simulink model "platoon_model"  (R2024a)
settings: Solver=VariableStepAuto  StartTime=0.0  StopTime=150  RelTol=1e-3
values from neighbouring files (symbols this model uses):
  d_0 = 8    [platoon.m]
  Kd_err = parameter_sets{i}.Kd_err    [platoon.m]
  Kv = parameter_sets{i}.Kv    [platoon.m]
  Kv_r = parameter_sets{i}.Kd_r    [platoon.m]
  t_h_tar = 1    [platoon.m]
  v_initial = v_initial_params{i}    [platoon.m]
  v_tar = 30    [platoon.m]
  x_initial = [150 100 50 0]    [platoon.m]
libraries: simulink x8
settings Model: Creator=alessandro  LastModifiedBy=vaidh
settings SolverCC: AlgebraicLoopSolver=TrustRegion
settings DebuggingCC: UnconnectedInputMsg=warning  UnconnectedOutputMsg=warning  UnconnectedLineMsg=warning
settings ModelReferenceCC: EnableRefExpFcnMdlSchedulingChecks=on
settings RTWCC: GPUComputeCapability=3.5  DLArmComputeVersion=19.05

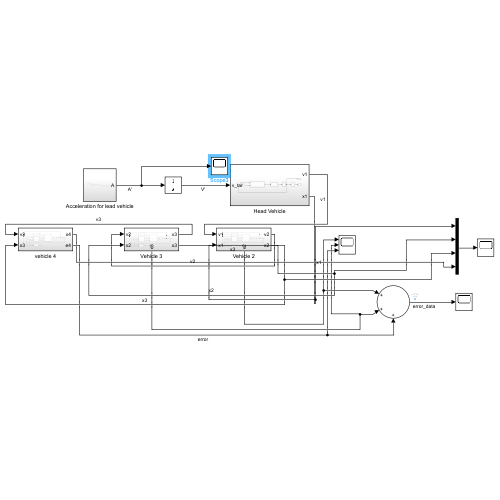
[thumbnail: Simulink's stored preview of the top-level diagram]
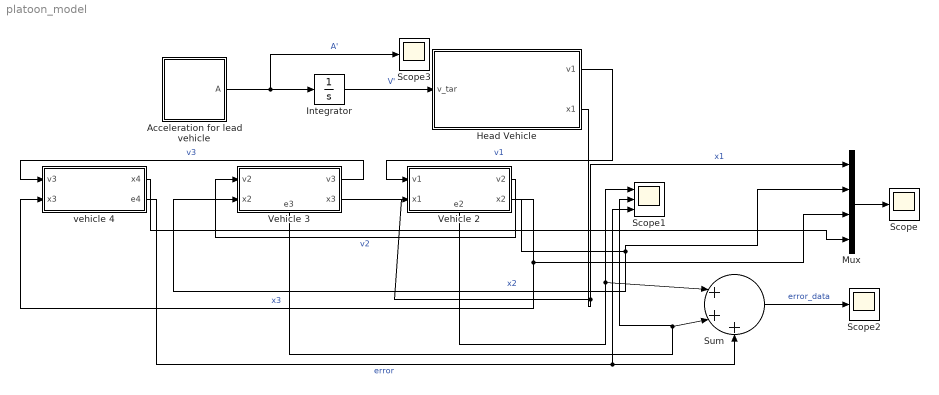
== system platoon_model ==
  Acceleration for lead vehicle : Subsystem
  "Head Vehicle " : Subsystem
  Integrator : Integrator  InitialCondition=v_initial(1)
  Mux : Mux
  Scope : Scope
  Scope1 : Scope  NumInputPorts=3
  Scope2 : Scope
  Scope3 : Scope
  Sum : Sum  Inputs=|+++
  Vehicle 2 : Subsystem
      settings: PortSchema="{\"entries\":[{\"content\":{\"sides\":[{\"content\":{\"connectorIds\":[\"In1\",\"In2\"]},\"type\":\"ConnectorPlacement.EquallySpacedRectSide\",\"uuid\":\"2c5fe078-c65f-41b6-8525-e64b013db54d\"},{\"content\":{\"connectorIds\":[\"Out1\",\"Out2\"],\"side\":\"RIGHT\"},\"type\":\"ConnectorPlacement.EquallySpacedRectSide\",\"uuid\":\"224ddbf7-34e7-4cd5-bbc2-438b58b736fb\"},{\"content\":{\"connectorIds\":[],\"side\":\"TOP\"},\"type\":\"ConnectorPlacement.EquallySpacedRectSide\",\"uuid\":\"73fb06e4-4483-4cd2-bdf8-037e0f1850b0\"},{\"content\":{\"connectorIds\":[\"Out3\"],\"side\":\"BOTTOM\"},\"type\":\"ConnectorPlacement.EquallySpacedRectSide\",\"uuid\":\"d300d9ad-fcb1-499a-b20a-481d5a2cf245\"},{\"content\":{\"connectorIds\":[],\"side\":\"HIDDEN\"},\"type\":\"ConnectorPlacement.EquallySpacedRectSide\",\"uuid\":\"4daeff91-7956-45e4-9a34-f5db9c954101\"}]},\"type\":\"ConnectorPlacement.EquallySpacedConnector\",\"uuid\":\"d1502d10-77ac-432c-94f4-53576a23d313\"}],\"packageUris\":[\"http://schema.mathworks.com/mf0/Connector/R2020b\"],\"version\":\"1.0\"}"
  Vehicle 3 : Subsystem
      settings: PortSchema="{\"entries\":[{\"content\":{\"sides\":[{\"content\":{\"connectorIds\":[\"In1\",\"In2\"]},\"type\":\"ConnectorPlacement.EquallySpacedRectSide\",\"uuid\":\"2c5fe078-c65f-41b6-8525-e64b013db54d\"},{\"content\":{\"connectorIds\":[\"Out1\",\"Out2\"],\"side\":\"RIGHT\"},\"type\":\"ConnectorPlacement.EquallySpacedRectSide\",\"uuid\":\"224ddbf7-34e7-4cd5-bbc2-438b58b736fb\"},{\"content\":{\"connectorIds\":[],\"side\":\"TOP\"},\"type\":\"ConnectorPlacement.EquallySpacedRectSide\",\"uuid\":\"73fb06e4-4483-4cd2-bdf8-037e0f1850b0\"},{\"content\":{\"connectorIds\":[\"Out3\"],\"side\":\"BOTTOM\"},\"type\":\"ConnectorPlacement.EquallySpacedRectSide\",\"uuid\":\"c04e4dd6-a406-4b84-b6be-e044dc5934f0\"},{\"content\":{\"connectorIds\":[],\"side\":\"HIDDEN\"},\"type\":\"ConnectorPlacement.EquallySpacedRectSide\",\"uuid\":\"4daeff91-7956-45e4-9a34-f5db9c954101\"}]},\"type\":\"ConnectorPlacement.EquallySpacedConnector\",\"uuid\":\"d1502d10-77ac-432c-94f4-53576a23d313\"}],\"packageUris\":[\"http://schema.mathworks.com/mf0/Connector/R2020b\"],\"version\":\"1.0\"}"
  vehicle 4 : Subsystem
  wires:
  Acceleration for lead vehicle/1(A) -> Scope3/1, Integrator/1  "A'"
  Integrator/1 -> "Head Vehicle "/1(v_tar)  "V'"
  "Head Vehicle "/1(v1) -> Vehicle 2/1(v1)  "v1"
  "Head Vehicle "/2(x1) -> Mux/1, Vehicle 2/2(x1)  "x1"
  Vehicle 2/1(v2) -> Vehicle 3/1(v2)  "v2"
  Vehicle 2/2(x2) -> Vehicle 3/2(x2), Mux/2  "x2"
  Vehicle 3/1(v3) -> vehicle 4/1(v3)  "v3"
  Vehicle 3/2(x3) -> vehicle 4/2(x3), Mux/3  "x3"
  vehicle 4/1(x4) -> Mux/4
  Mux/1 -> Scope/1
  Vehicle 3/3(e3) -> Sum/2, Scope1/2
  Vehicle 2/3(e2) -> Sum/1, Scope1/1
  vehicle 4/2(e4) -> Sum/3, Scope1/3  "error"
  Sum/1 -> Scope2/1  "error_data"

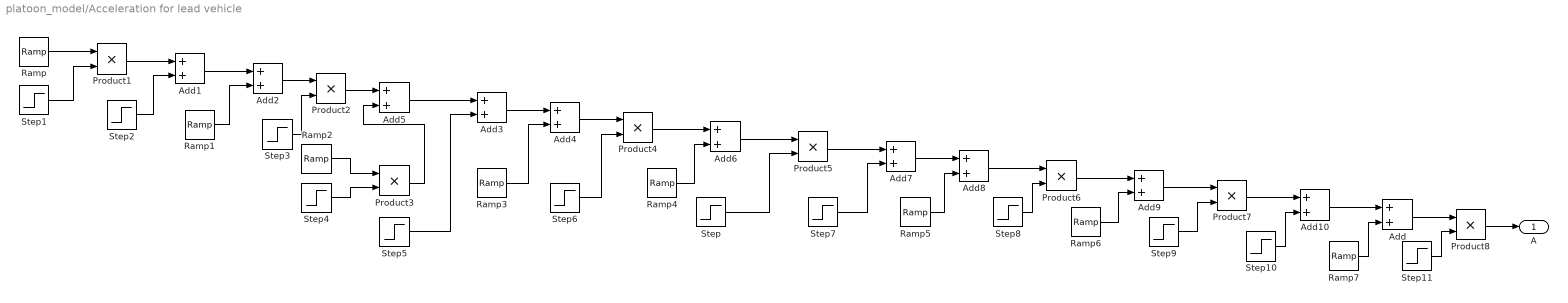
== system platoon_model/Acceleration for lead vehicle ==
  Add{,1..10} (11 alike) : Sum
  Product{1..8} (8 alike) : Product
  Ramp : simulink/Sources/Ramp  slope=-4  start=10  InitialOutput=0
  Ramp1 : simulink/Sources/Ramp  slope=4  start=13.5  InitialOutput=0
  Ramp2 : simulink/Sources/Ramp  slope=4  start=40  InitialOutput=0
  Ramp3 : simulink/Sources/Ramp  slope=-4  start=43.5  InitialOutput=0
  Ramp4 : simulink/Sources/Ramp  slope=-4  start=70  InitialOutput=0
  Ramp5 : simulink/Sources/Ramp  slope=4  start=73.5  InitialOutput=0
  Ramp6 : simulink/Sources/Ramp  slope=4  start=100  InitialOutput=0
  Ramp7 : simulink/Sources/Ramp  slope=-4  start=103.5  InitialOutput=0
  Step : Step  Time=70.5  Before=1  After=0  SampleTime=0
  Step1 : Step  Time=10.5  Before=1  After=0  SampleTime=0.1
  Step10 : Step  Time=100.5  After=2  SampleTime=0
  Step11 : Step  Time=104  Before=1  After=0  SampleTime=0
  Step2 : Step  Time=10.5  After=-2  SampleTime=0
  Step3 : Step  Time=14  Before=1  After=0  SampleTime=0
  Step4 : Step  Time=40.5  Before=1  After=0  SampleTime=0
  Step5 : Step  Time=40.5  After=2  SampleTime=0
  Step6 : Step  Time=44  Before=1  After=0  SampleTime=0
  Step7 : Step  Time=70.5  After=-2  SampleTime=0
  Step8 : Step  Time=74  Before=1  After=0  SampleTime=0
  Step9 : Step  Time=100.5  Before=1  After=0  SampleTime=0
  A : Outport
  wires:
  Add1/1 -> Add2/1
  Step3/1 -> Product2/2
  Product3/1 -> Add5/2
  Step5/1 -> Add3/2
  Add2/1 -> Product2/1
  Step1/1 -> Product1/2
  Product2/1 -> Add5/1
  Step2/1 -> Add1/2
  Ramp2/1 -> Product3/1
  Product1/1 -> Add1/1
  Add4/1 -> Product4/1
  Ramp/1 -> Product1/1
  Add3/1 -> Add4/1
  Step6/1 -> Product4/2
  Ramp1/1 -> Add2/2
  Step4/1 -> Product3/2
  Add5/1 -> Add3/1
  Ramp3/1 -> Add4/2
  Product4/1 -> Add6/1
  Ramp4/1 -> Add6/2
  Add6/1 -> Product5/1
  Step/1 -> Product5/2
  Product5/1 -> Add7/1
  Step7/1 -> Add7/2
  Add7/1 -> Add8/1
  Ramp5/1 -> Add8/2
  Add8/1 -> Product6/1
  Step8/1 -> Product6/2
  Product6/1 -> Add9/1
  Ramp6/1 -> Add9/2
  Add9/1 -> Product7/1
  Step9/1 -> Product7/2
  Step10/1 -> Add10/2
  Product7/1 -> Add10/1
  Add10/1 -> Add/1
  Ramp7/1 -> Add/2
  Add/1 -> Product8/1
  Step11/1 -> Product8/2
  Product8/1 -> A/1

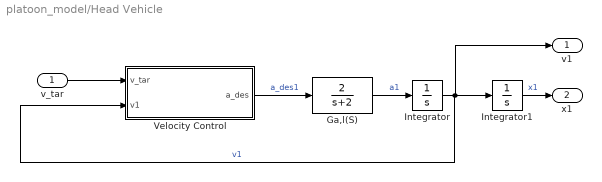
== system platoon_model/Head Vehicle  ==
  v_tar : Inport
  Ga,l(S) : TransferFcn  Numerator=[2]  Denominator=[1 2]
  Integrator : Integrator  InitialCondition=v_initial(1)
  Integrator1 : Integrator  InitialCondition=x_initial(1)
  Velocity Control : Subsystem
  v1 : Outport
  x1 : Outport  Port=2
  wires:
  Integrator/1 -> Velocity Control/2(v1), v1/1, Integrator1/1  "v1"
  Ga,l(S)/1 -> Integrator/1  "a1"
  v_tar/1 -> Velocity Control/1(v_tar)
  Velocity Control/1(a_des) -> Ga,l(S)/1  "a_des1"
  Integrator1/1 -> x1/1  "x1"

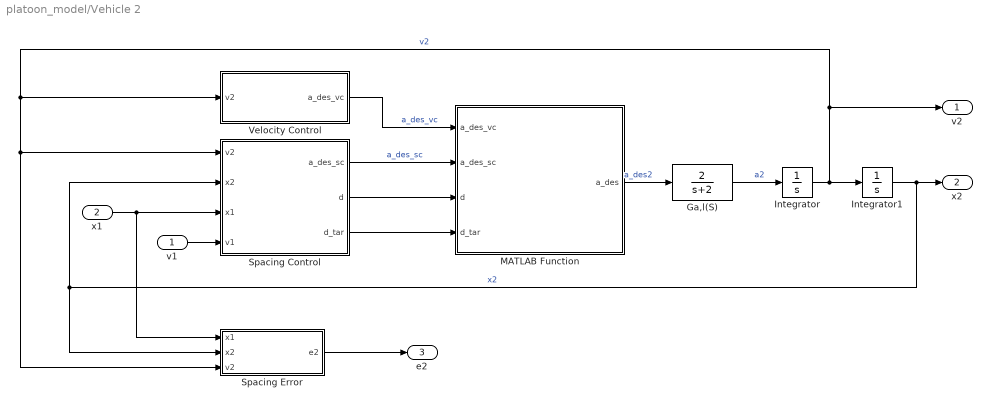
== system platoon_model/Vehicle 2 ==
  v1 : Inport
  x1 : Inport  Port=2
  Ga,l(S) : TransferFcn  Numerator=[2]  Denominator=[1 2]
  Integrator : Integrator  InitialCondition=v_initial(2)
  Integrator1 : Integrator  InitialCondition=x_initial(2)
  MATLAB Function : MATLAB Function  TreatAsAtomicUnit=on
  Spacing Control : Subsystem
  Spacing Error : Subsystem
  Velocity Control : Subsystem
  v2 : Outport
  x2 : Outport  Port=2
  e2 : Outport  Port=3
  wires:
  Spacing Control/1(a_des_sc) -> MATLAB Function/2(a_des_sc)  "a_des_sc"
  Velocity Control/1(a_des_vc) -> MATLAB Function/1(a_des_vc)  "a_des_vc"
  v1/1 -> Spacing Control/4(v1)
  x1/1 -> Spacing Control/3(x1), Spacing Error/1(x1)
  Spacing Control/2(d) -> MATLAB Function/3(d)
  MATLAB Function/1(a_des) -> Ga,l(S)/1  "a_des2"
  Integrator1/1 -> x2/1, Spacing Error/2(x2), Spacing Control/2(x2)  "x2"
  Spacing Control/3(d_tar) -> MATLAB Function/4(d_tar)
  Ga,l(S)/1 -> Integrator/1  "a2"
  Integrator/1 -> Integrator1/1, v2/1, Velocity Control/1(v2), Spacing Control/1(v2), Spacing Error/3(v2)  "v2"
  Spacing Error/1(e2) -> e2/1

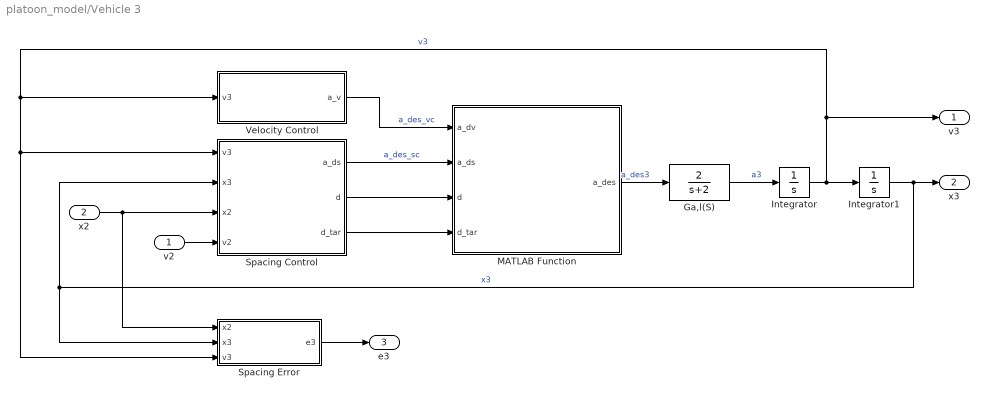
== system platoon_model/Vehicle 3 ==
  v2 : Inport
  x2 : Inport  Port=2
  Ga,l(S) : TransferFcn  Numerator=[2]  Denominator=[1 2]
  Integrator : Integrator  InitialCondition=v_initial(3)
  Integrator1 : Integrator  InitialCondition=x_initial(3)
  MATLAB Function : MATLAB Function  TreatAsAtomicUnit=on
  Spacing Control : Subsystem
  Spacing Error : Subsystem
  Velocity Control : Subsystem
  v3 : Outport
  x3 : Outport  Port=2
  e3 : Outport  Port=3
  wires:
  Spacing Control/1(a_ds) -> MATLAB Function/2(a_ds)  "a_des_sc"
  Velocity Control/1(a_v) -> MATLAB Function/1(a_dv)  "a_des_vc"
  v2/1 -> Spacing Control/4(v2)
  x2/1 -> Spacing Error/1(x2), Spacing Control/3(x2)
  Spacing Control/2(d) -> MATLAB Function/3(d)
  MATLAB Function/1(a_des) -> Ga,l(S)/1  "a_des3"
  Integrator1/1 -> x3/1, Spacing Error/2(x3), Spacing Control/2(x3)  "x3"
  Spacing Control/3(d_tar) -> MATLAB Function/4(d_tar)
  Ga,l(S)/1 -> Integrator/1  "a3"
  Integrator/1 -> Integrator1/1, v3/1, Velocity Control/1(v3), Spacing Error/3(v3), Spacing Control/1(v3)  "v3"
  Spacing Error/1(e3) -> e3/1

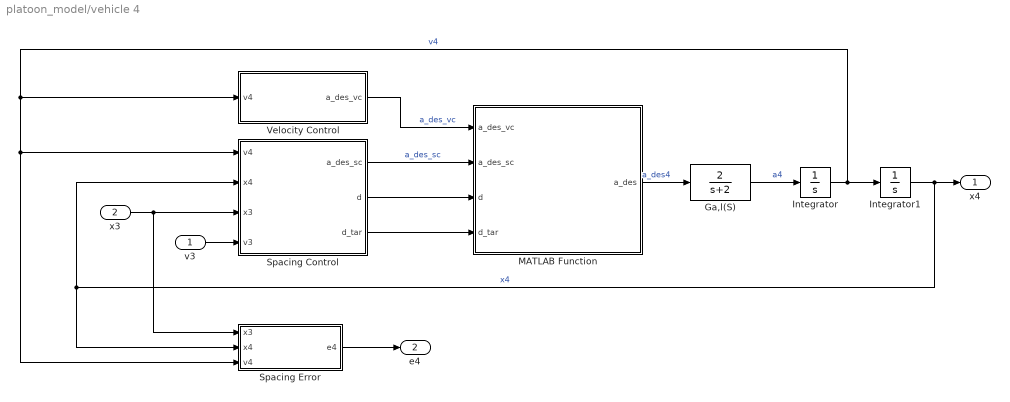
== system platoon_model/vehicle 4 ==
  v3 : Inport
  x3 : Inport  Port=2
  Ga,l(S) : TransferFcn  Numerator=[2]  Denominator=[1 2]
  Integrator : Integrator  InitialCondition=v_initial(4)
  Integrator1 : Integrator  InitialCondition=x_initial(4)
  MATLAB Function : MATLAB Function  TreatAsAtomicUnit=on
  Spacing Control : Subsystem
  Spacing Error : Subsystem
  Velocity Control : Subsystem
  x4 : Outport
  e4 : Outport  Port=2
  wires:
  Spacing Control/1(a_des_sc) -> MATLAB Function/2(a_des_sc)  "a_des_sc"
  Velocity Control/1(a_des_vc) -> MATLAB Function/1(a_des_vc)  "a_des_vc"
  v3/1 -> Spacing Control/4(v3)
  x3/1 -> Spacing Error/1(x3), Spacing Control/3(x3)
  Spacing Control/2(d) -> MATLAB Function/3(d)
  MATLAB Function/1(a_des) -> Ga,l(S)/1  "a_des4"
  Integrator1/1 -> x4/1, Spacing Error/2(x4), Spacing Control/2(x4)  "x4"
  Spacing Control/3(d_tar) -> MATLAB Function/4(d_tar)
  Ga,l(S)/1 -> Integrator/1  "a4"
  Integrator/1 -> Integrator1/1, Velocity Control/1(v4), Spacing Error/3(v4), Spacing Control/1(v4)  "v4"
  Spacing Error/1(e4) -> e4/1

== system platoon_model/Head Vehicle /Velocity Control ==
  v_tar : Inport
  v1 : Inport  Port=2
  Gain : Gain  Gain=Kv
  Subtract : Sum  Inputs=+-
  a_des : Outport
  wires:
  v1/1 -> Subtract/2
  v_tar/1 -> Subtract/1
  Subtract/1 -> Gain/1  "e_v"
  Gain/1 -> a_des/1  "a_des"

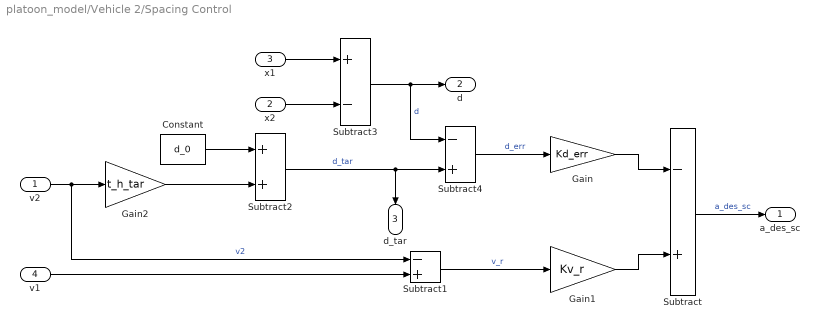
== system platoon_model/Vehicle 2/Spacing Control ==
  v2 : Inport
  x2 : Inport  Port=2
  x1 : Inport  Port=3
  v1 : Inport  Port=4
  Constant : Constant  Value=d_0
  Gain : Gain  Gain=Kd_err
  Gain1 : Gain  Gain=Kv_r
  Gain2 : Gain  Gain=t_h_tar
  Subtract : Sum  Inputs=-+
  Subtract1 : Sum  Inputs=-+
  Subtract2 : Sum
  Subtract3 : Sum  Inputs=+-
  Subtract4 : Sum  Inputs=-+
  a_des_sc : Outport
  d : Outport  Port=2
  d_tar : Outport  Port=3
  wires:
  Gain/1 -> Subtract/1
  Gain1/1 -> Subtract/2
  Subtract/1 -> a_des_sc/1  "a_des_sc"
  v2/1 -> Subtract1/1, Gain2/1  "v2"
  Subtract1/1 -> Gain1/1  "v_r"
  Gain2/1 -> Subtract2/2
  v1/1 -> Subtract1/2
  x1/1 -> Subtract3/1
  x2/1 -> Subtract3/2
  Subtract2/1 -> Subtract4/2, d_tar/1  "d_tar"
  Subtract3/1 -> Subtract4/1, d/1  "d"
  Subtract4/1 -> Gain/1  "d_err"
  Constant/1 -> Subtract2/1

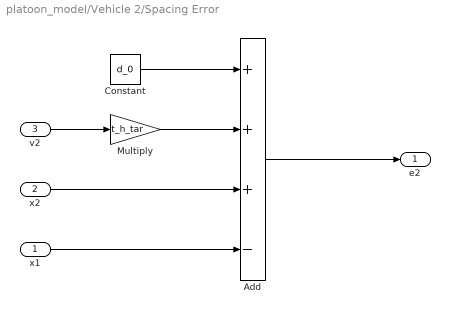
== system platoon_model/Vehicle 2/Spacing Error ==
  x1 : Inport
  x2 : Inport  Port=2
  v2 : Inport  Port=3
  Add : Sum  Inputs=+++-
  Constant : Constant  Value=d_0
  Multiply : Gain  Gain=t_h_tar
  e2 : Outport
  wires:
  Constant/1 -> Add/1
  Multiply/1 -> Add/2
  v2/1 -> Multiply/1
  x2/1 -> Add/3
  x1/1 -> Add/4
  Add/1 -> e2/1

== system platoon_model/Vehicle 2/Velocity Control ==
  v2 : Inport
  Constant : Constant  Value=v_tar
  Gain : Gain  Gain=Kv
  Subtract : Sum  Inputs=+-
  a_des_vc : Outport
  wires:
  v2/1 -> Subtract/2
  Constant/1 -> Subtract/1
  Subtract/1 -> Gain/1  "e_v"
  Gain/1 -> a_des_vc/1  "a_des_vc"

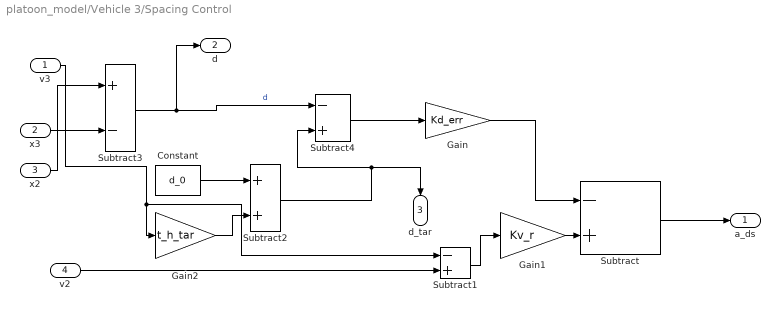
== system platoon_model/Vehicle 3/Spacing Control ==
  v3 : Inport
  x3 : Inport  Port=2
  x2 : Inport  Port=3
  v2 : Inport  Port=4
  Constant : Constant  Value=d_0
  Gain : Gain  Gain=Kd_err
  Gain1 : Gain  Gain=Kv_r
  Gain2 : Gain  Gain=t_h_tar
  Subtract : Sum  Inputs=-+
  Subtract1 : Sum  Inputs=-+
  Subtract2 : Sum
  Subtract3 : Sum  Inputs=+-
  Subtract4 : Sum  Inputs=-+
  a_ds : Outport
  d : Outport  Port=2
  d_tar : Outport  Port=3
  wires:
  Gain/1 -> Subtract/1
  Gain1/1 -> Subtract/2
  Subtract/1 -> a_ds/1
  v3/1 -> Subtract1/1, Gain2/1
  Subtract1/1 -> Gain1/1
  Gain2/1 -> Subtract2/2
  v2/1 -> Subtract1/2
  x2/1 -> Subtract3/1
  x3/1 -> Subtract3/2
  Subtract2/1 -> d_tar/1, Subtract4/2
  Subtract3/1 -> Subtract4/1, d/1  "d"
  Subtract4/1 -> Gain/1
  Constant/1 -> Subtract2/1

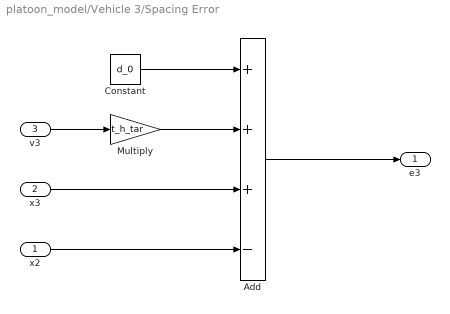
== system platoon_model/Vehicle 3/Spacing Error ==
  x2 : Inport
  x3 : Inport  Port=2
  v3 : Inport  Port=3
  Add : Sum  Inputs=+++-
  Constant : Constant  Value=d_0
  Multiply : Gain  Gain=t_h_tar
  e3 : Outport
  wires:
  Constant/1 -> Add/1
  Multiply/1 -> Add/2
  v3/1 -> Multiply/1
  x3/1 -> Add/3
  x2/1 -> Add/4
  Add/1 -> e3/1

== system platoon_model/Vehicle 3/Velocity Control ==
  v3 : Inport
  Constant : Constant  Value=v_tar
  Gain : Gain  Gain=Kv
  Subtract : Sum  Inputs=+-
  a_v : Outport
  wires:
  v3/1 -> Subtract/2
  Constant/1 -> Subtract/1
  Subtract/1 -> Gain/1
  Gain/1 -> a_v/1

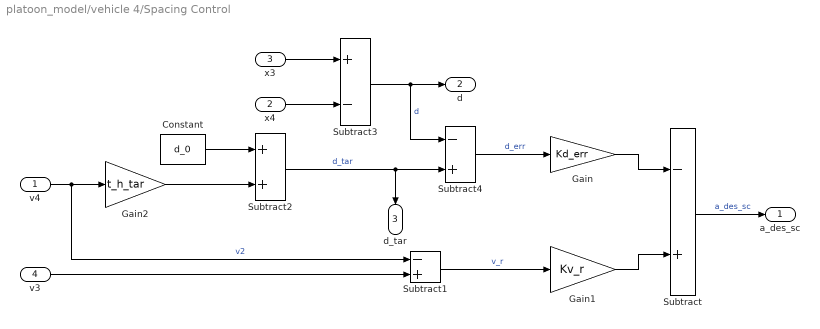
== system platoon_model/vehicle 4/Spacing Control ==
  v4 : Inport
  x4 : Inport  Port=2
  x3 : Inport  Port=3
  v3 : Inport  Port=4
  Constant : Constant  Value=d_0
  Gain : Gain  Gain=Kd_err
  Gain1 : Gain  Gain=Kv_r
  Gain2 : Gain  Gain=t_h_tar
  Subtract : Sum  Inputs=-+
  Subtract1 : Sum  Inputs=-+
  Subtract2 : Sum
  Subtract3 : Sum  Inputs=+-
  Subtract4 : Sum  Inputs=-+
  a_des_sc : Outport
  d : Outport  Port=2
  d_tar : Outport  Port=3
  wires:
  Gain/1 -> Subtract/1
  Gain1/1 -> Subtract/2
  Subtract/1 -> a_des_sc/1  "a_des_sc"
  v4/1 -> Subtract1/1, Gain2/1  "v2"
  Subtract1/1 -> Gain1/1  "v_r"
  Gain2/1 -> Subtract2/2
  v3/1 -> Subtract1/2
  x3/1 -> Subtract3/1
  x4/1 -> Subtract3/2
  Subtract2/1 -> Subtract4/2, d_tar/1  "d_tar"
  Subtract3/1 -> Subtract4/1, d/1  "d"
  Subtract4/1 -> Gain/1  "d_err"
  Constant/1 -> Subtract2/1

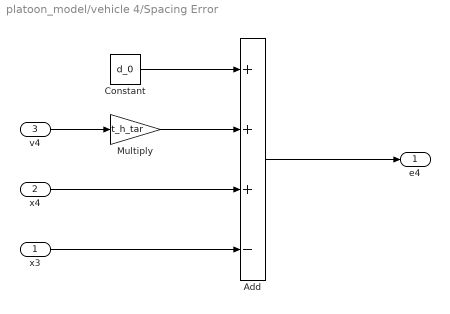
== system platoon_model/vehicle 4/Spacing Error ==
  x3 : Inport
  x4 : Inport  Port=2
  v4 : Inport  Port=3
  Add : Sum  Inputs=+++-
  Constant : Constant  Value=d_0
  Multiply : Gain  Gain=t_h_tar
  e4 : Outport
  wires:
  Constant/1 -> Add/1
  Multiply/1 -> Add/2
  v4/1 -> Multiply/1
  x4/1 -> Add/3
  x3/1 -> Add/4
  Add/1 -> e4/1

== system platoon_model/vehicle 4/Velocity Control ==
  v4 : Inport
  Constant : Constant  Value=v_tar
  Gain : Gain  Gain=Kv
  Subtract : Sum  Inputs=+-
  a_des_vc : Outport
  wires:
  v4/1 -> Subtract/2
  Constant/1 -> Subtract/1
  Subtract/1 -> Gain/1  "e_v"
  Gain/1 -> a_des_vc/1  "a_des_vc"

== matlab function platoon_model/Vehicle 2/MATLAB Function ==
  data: a_des_vc input; a_des output; a_des_sc input; d input; d_tar input
function a_des = switching_logic(a_des_vc, a_des_sc, d, d_tar)

if d > d_tar
    a_des = min([a_des_vc a_des_sc]);
else
    a_des = a_des_sc;
end

if a_des > 5 
    a_des = 5;
end

if a_des < -3
    a_des = -3;
end


end

== matlab function platoon_model/Vehicle 3/MATLAB Function ==
  data: a_dv input; a_des output; a_ds input; d input; d_tar input
function a_des = switching_logic(a_dv, a_ds, d, d_tar)

if d > d_tar
    a_des = min([a_dv a_ds]);
else
    a_des = a_ds;
end

if a_des > 5 
    a_des = 5;
end

if a_des < -3
    a_des = -3;
end


end

== matlab function platoon_model/vehicle 4/MATLAB Function ==
  data: a_des_vc input; a_des output; a_des_sc input; d input; d_tar input
function a_des = switching_logic(a_des_vc, a_des_sc, d, d_tar)

if d > d_tar
    a_des = min([a_des_vc a_des_sc]);
else
    a_des = a_des_sc;
end

if a_des > 5 
    a_des = 5;
end

if a_des < -3
    a_des = -3;
end


end
